simulink subsystem "eomModel"  (R2026a)
settings: Solver=VariableStepAuto
values from neighbouring files (symbols this model uses):
  vehicleParams = 18.0    [plantParams.sldd]
libraries: aerolib6dof2 x2
settings Model: DataDictionary=plantParams.sldd  EnableAccessToBaseWorkspace=off  Creator=maxhu  LastModifiedBy=maxhu

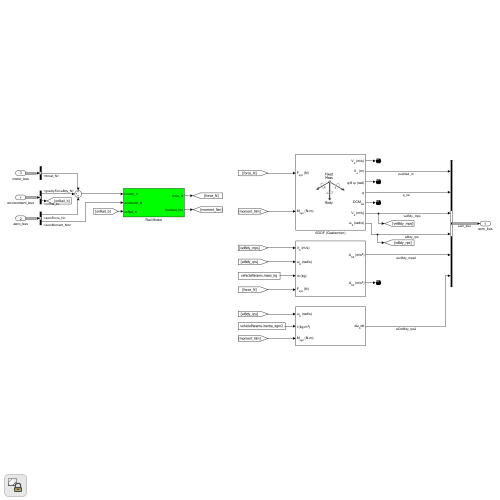
[thumbnail: Simulink's stored preview of the top-level diagram]
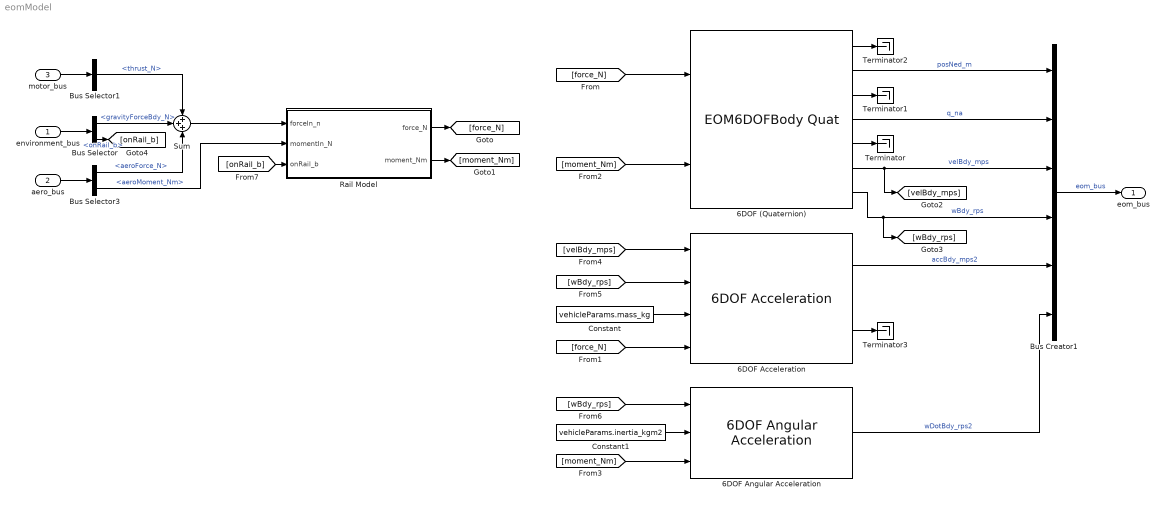
== system eomModel ==
  environment_bus : Inport
  aero_bus : Inport  Port=2
  motor_bus : Inport  Port=3
  6DOF (Quaternion) : EOM6DOFBodyQuat  xme_0=icParams.posNed_m  Vm_0=icParams.velBdy_mps  eul_0=icParams.eul_rad  pm_0=icParams.rateBdy_rps  mass_0=vehicleParams.mass_kg  inertia=vehicleParams.inertia_kgm2
  6DOF Acceleration : aerolib6dof2/6DOF Acceleration  units=Metric (MKS)  mtype=Fixed  vre_flag=off
  6DOF Angular Acceleration : aerolib6dof2/6DOF Angular Acceleration  units=Metric (MKS)  mtype=Fixed
  Bus Creator1 : BusCreator  Inputs=6
  Bus Selector : BusSelector  OutputSignals=gravityForceBdy_N,onRail_b
  Bus Selector1 : BusSelector  OutputSignals=thrust_N
  Bus Selector3 : BusSelector  OutputSignals=aeroForce_N,aeroMoment_Nm
  Constant : Constant  Value=vehicleParams.mass_kg
  Constant1 : Constant  Value=vehicleParams.inertia_kgm2
  Rail Model : Subsystem
  Sum : Sum  Inputs=+++
  Terminator{,1..3} (4 alike) : Terminator
  eom_bus : Outport
  wires:
  6DOF (Quaternion)/3 -> Terminator1/1
  6DOF (Quaternion)/6 -> Bus Creator1/3, [velBdy_mps]  "velBdy_mps"
  6DOF (Quaternion)/2 -> Bus Creator1/1  "posNed_m"
  6DOF (Quaternion)/1 -> Terminator2/1
  6DOF (Quaternion)/5 -> Terminator/1
  6DOF (Quaternion)/7 -> Bus Creator1/4, [wBdy_rps]  "wBdy_rps"
  6DOF (Quaternion)/4 -> Bus Creator1/2  "q_na"
  Bus Creator1/1 -> eom_bus/1  "eom_bus"
  environment_bus/1 -> Bus Selector/1
  aero_bus/1 -> Bus Selector3/1
  6DOF Acceleration/2 -> Terminator3/1
  6DOF Acceleration/1 -> Bus Creator1/5  "accBdy_mps2"
  6DOF Angular Acceleration/1 -> Bus Creator1/6  "wDotBdy_rps2"
  Constant/1 -> 6DOF Acceleration/3
  Constant1/1 -> 6DOF Angular Acceleration/2
  [force_N] -> 6DOF (Quaternion)/1
  [force_N] -> 6DOF Acceleration/4
  [moment_Nm] -> 6DOF Angular Acceleration/3
  [velBdy_mps] -> 6DOF Acceleration/1
  [wBdy_rps] -> 6DOF Acceleration/2
  [wBdy_rps] -> 6DOF Angular Acceleration/1
  Bus Selector3/1 -> Sum/3  "<aeroForce_N>"
  Bus Selector/1 -> Sum/2  "<gravityForceBdy_N>"
  motor_bus/1 -> Bus Selector1/1
  Bus Selector1/1 -> Sum/1  "<thrust_N>"
  [moment_Nm] -> 6DOF (Quaternion)/2
  Sum/1 -> Rail Model/1(forceIn_n)
  Bus Selector3/2 -> Rail Model/2(momentIn_N)  "<aeroMoment_Nm>"
  Rail Model/1(force_N) -> [force_N]
  Rail Model/2(moment_Nm) -> [moment_Nm]
  Bus Selector/2 -> [onRail_b]  "<onRail_b>"
  [onRail_b] -> Rail Model/3(onRail_b)

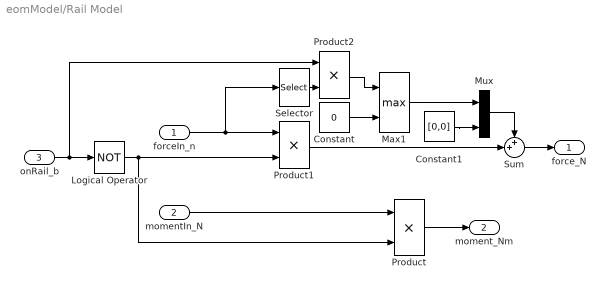
== system eomModel/Rail Model ==
  forceIn_n : Inport
  momentIn_N : Inport  Port=2
  onRail_b : Inport  Port=3
  Constant : Constant  Value=0
  Constant1 : Constant  Value=[0,0]
  Logical Operator : Logic  Operator=NOT  AllPortsSameDT=off  OutDataTypeStr=boolean
  Max1 : MinMax  Function=max  Inputs=2
  Mux : Mux  Inputs=2
  Product : Product
  Product1 : Product
  Product2 : Product
  Selector : Selector  InputPortWidth=3  IndexOptions=Index vector (dialog)  Indices=[1]  OutputSizes=1
  Sum : Sum  Inputs=++|
  force_N : Outport
  moment_Nm : Outport  Port=2
  wires:
  Product2/1 -> Max1/1
  Selector/1 -> Product2/2
  Constant/1 -> Max1/2
  Logical Operator/1 -> Product/2, Product1/2
  momentIn_N/1 -> Product/1
  forceIn_n/1 -> Product1/1, Selector/1
  Product/1 -> moment_Nm/1
  onRail_b/1 -> Logical Operator/1, Product2/1
  Sum/1 -> force_N/1
  Product1/1 -> Sum/2
  Max1/1 -> Mux/1
  Constant1/1 -> Mux/2
  Mux/1 -> Sum/1
